simulink model "sampleModel1418"  (R2023a)
settings: Solver=VariableStepAuto  StartTime=0.0  StopTime=10.0  RelTol=1e-3
libraries: hdlsllib x5, simulink x2
settings Model: Creator=user1  LastModifiedBy=user1

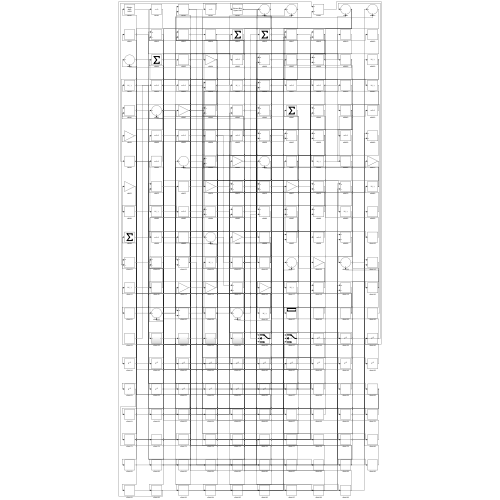
[thumbnail: Simulink's stored preview of the top-level diagram]
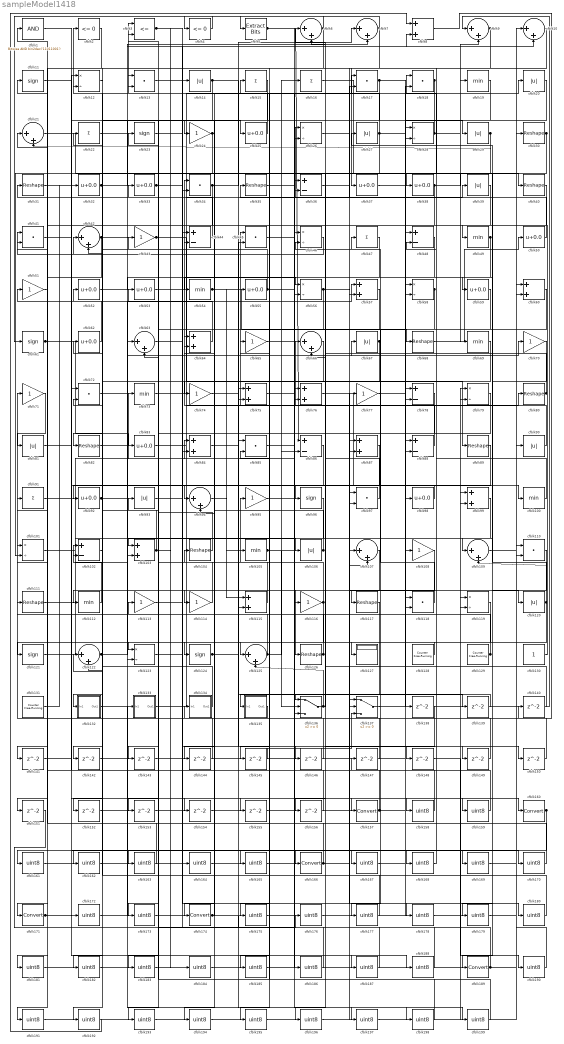
== system sampleModel1418 ==
  cfblk1 : simulink/Logic and Bit Operations/Bitwise Operator  logicop=AND  UseBitMask=on  BitMask=bin2dec('11011001')  BitMaskRealWorld=Stored Integer
      settings: LibrarySourceBlock=|
      | hdlsllib/Logic and Bit
      | Operations/Bitwise
      | Operator
  cfblk{6..7,9..10,21,42,63,66,94,107,109,122,125} (13 alike) : Sum  Inputs=|++
  cfblk{19,49,54,69,73,100,105,112} (8 alike) : MinMax
  cfblk{12,26,28,46,56,58,79,101,119,123} (10 alike) : Product  Inputs=*/  RndMeth=Zero  SaturateOnIntegerOverflow=on
  cfblk{36,44,48,78,86,88,102} (7 alike) : Sum  Inputs=+-
  cfblk{8,57,60,64,75..76,84,87,99,103,115} (11 alike) : Sum
  cfblk{30..31,35,40,68,80,82,89,104,111,117,126} (12 alike) : Reshape
  cfblk{14,20,27,29,39,67,81,90,93,106,120} (11 alike) : Abs  SaturateOnIntegerOverflow=off
  cfblk{24,43,51,65,70..71,74,77,95,108,113..114,116} (13 alike) : Gain
  cfblk{11,23,61,96,121,124} (6 alike) : Signum
  cfblk{13,17..18,34,41,45,72,85,97,110,118} (11 alike) : DotProduct  OutDataTypeStr=Inherit: Inherit via internal rule
  cfblk127 : Display
  cfblk128 : hdlsllib/Sources/Counter Free-Running  NumBits=16  tsamp=-1
  cfblk129 : hdlsllib/Sources/Counter Free-Running  NumBits=16  tsamp=-1
  cfblk130 : Constant  SampleTime=-1
  cfblk131 : hdlsllib/Sources/Counter Free-Running  NumBits=16  tsamp=-1
  cfblk132 : Subsystem
      settings: LibrarySourceBlock=|
      | hdlsllib/Ports &
      | Subsystems/Subsystem
  cfblk133 : Subsystem
      settings: LibrarySourceBlock=|
      | hdlsllib/Ports &
      | Subsystems/Subsystem
  cfblk134 : Subsystem
      settings: LibrarySourceBlock=|
      | hdlsllib/Ports &
      | Subsystems/Subsystem
  cfblk135 : Subsystem
      settings: LibrarySourceBlock=|
      | hdlsllib/Ports &
      | Subsystems/Subsystem
  cfblk136 : Switch  SaturateOnIntegerOverflow=off  InputSameDT=off
  cfblk137 : Switch  SaturateOnIntegerOverflow=off  InputSameDT=off
  cfblk{138..156} (19 alike) : Delay  SampleTime=1
  cfblk{15..16,22,47,91} (5 alike) : Sum  Inputs=+
  cfblk{157,160,166,171,174,189} (6 alike) : DataTypeConversion  SaturateOnIntegerOverflow=off  RndMeth=Floor
  cfblk{158..159,161..165,167..170,172..173,175..188,190..199} (37 alike) : DataTypeConversion  OutDataTypeStr=uint8  SaturateOnIntegerOverflow=off  RndMeth=Floor
  cfblk2 : hdlsllib/Logic and Bit Operations/Compare To Zero  relop=<=  OutDataTypeStr=boolean
  cfblk{25,32..33,37..38,50,52..53,55,59,62,83,92,98} (14 alike) : Bias  Bias=0.0  SaturateOnIntegerOverflow=off
  cfblk3 : RelationalOperator  Operator=<=  OutDataTypeStr=boolean  InputSameDT=off
  cfblk4 : hdlsllib/Logic and Bit Operations/Compare To Zero  relop=<=  OutDataTypeStr=boolean
  cfblk5 : simulink/Logic and Bit Operations/Extract Bits  bitsToExtract=Upper half  numBits=8  bitIdxRange=[0 7]  outScalingMode=Preserve fixed-point scaling
      settings: LibrarySourceBlock=|
      | hdlsllib/Logic and Bit
      | Operations/Extract Bits
  wires:
  cfblk73/1 -> cfblk20/1
  cfblk94/1 -> cfblk115/1
  cfblk68/1 -> cfblk50/1
  cfblk42/1 -> cfblk56/2, cfblk151/1, cfblk170/1
  cfblk130/1 -> cfblk49/1
  cfblk88/1 -> cfblk45/1
  cfblk25/1 -> cfblk2/1
  cfblk106/1 -> cfblk15/1, cfblk13/1
  cfblk54/1 -> cfblk68/1, cfblk105/1
  cfblk83/1 -> cfblk39/1
  cfblk131/1 -> cfblk32/1
  cfblk15/1 -> cfblk82/1
  cfblk121/1 -> cfblk73/1
  cfblk1/1 -> cfblk25/1
  cfblk90/1 -> cfblk34/1
  cfblk93/1 -> cfblk14/1
  cfblk104/1 -> cfblk53/1
  cfblk5/1 -> cfblk86/1, cfblk40/1
  cfblk97/1 -> cfblk6/1
  cfblk135/1(Out1) -> cfblk71/1
  cfblk19/1 -> cfblk74/1
  cfblk101/1 -> cfblk106/1
  cfblk9/1 -> cfblk37/1, cfblk122/2, cfblk57/2
  cfblk18/1 -> cfblk28/2, cfblk103/2
  cfblk12/1 -> cfblk42/2
  cfblk110/1 -> cfblk189/1
  cfblk112/1 -> cfblk102/1
  cfblk80/1 -> cfblk35/1, cfblk47/1
  cfblk28/1 -> cfblk24/1, cfblk9/2
  cfblk117/1 -> cfblk135/1(In1)
  cfblk100/1 -> cfblk18/1
  cfblk61/1 -> cfblk83/1, cfblk187/1
  cfblk34/1 -> cfblk7/1, cfblk123/2
  cfblk57/1 -> cfblk115/2
  cfblk119/1 -> cfblk171/1
  cfblk75/1 -> cfblk160/1
  cfblk7/1 -> cfblk5/1, cfblk152/1
  cfblk108/1 -> cfblk126/1
  cfblk55/1 -> cfblk31/1, cfblk13/2, cfblk159/1
  cfblk70/1 -> cfblk109/1
  cfblk115/1 -> cfblk95/1
  cfblk16/1 -> cfblk98/1
  cfblk133/1(Out1) -> cfblk66/1
  cfblk21/1 -> cfblk69/1
  cfblk96/1 -> cfblk123/1
  cfblk91/1 -> cfblk46/1
  cfblk58/1 -> cfblk124/1, cfblk117/1
  cfblk86/1 -> cfblk125/1
  cfblk52/1 -> cfblk56/1
  cfblk125/1 -> cfblk41/1, cfblk16/1
  cfblk72/1 -> cfblk157/1
  cfblk4/1 -> cfblk61/1
  cfblk48/1 -> cfblk166/1
  cfblk82/1 -> cfblk67/1
  cfblk62/1 -> cfblk11/1
  cfblk56/1 -> cfblk94/1, cfblk150/1
  cfblk124/1 -> cfblk80/1, cfblk194/1
  cfblk118/1 -> cfblk46/2
  cfblk122/1 -> cfblk70/1, cfblk55/1
  cfblk32/1 -> cfblk7/2, cfblk182/1
  cfblk47/1 -> cfblk94/2
  cfblk120/1 -> cfblk27/1, cfblk109/2, cfblk165/1
  cfblk27/1 -> cfblk29/1, cfblk103/1, cfblk3/2, cfblk101/2
  cfblk6/1 -> cfblk4/1, cfblk175/1
  cfblk23/1 -> cfblk34/2
  cfblk71/1 -> cfblk81/1
  cfblk116/1 -> cfblk44/2, cfblk161/1
  cfblk14/1 -> cfblk139/1, cfblk173/1
  cfblk78/1 -> cfblk174/1
  cfblk24/1 -> cfblk132/1(In1), cfblk54/1
  cfblk26/1 -> cfblk120/1
  cfblk50/1 -> cfblk26/1
  cfblk136/1 -> cfblk6/2, cfblk125/2
  cfblk74/1 -> cfblk57/1
  cfblk111/1 -> cfblk63/1
  cfblk33/1 -> cfblk143/1, cfblk167/1
  cfblk2/1 -> cfblk121/1
  cfblk76/1 -> cfblk108/1
  cfblk109/1 -> cfblk30/1
  cfblk92/1 -> cfblk84/1, cfblk112/1
  cfblk98/1 -> cfblk92/1
  cfblk77/1 -> cfblk118/1
  cfblk29/1 -> cfblk116/1, cfblk21/2
  cfblk43/1 -> cfblk89/1, cfblk17/2
  cfblk44/1 -> cfblk12/2
  cfblk103/1 -> cfblk52/1, cfblk184/1
  cfblk123/1 -> cfblk84/2
  cfblk53/1 -> cfblk97/2
  cfblk105/1 -> cfblk26/2, cfblk86/2, cfblk136/2
  cfblk45/1 -> cfblk100/1
  cfblk46/1 -> cfblk41/2
  cfblk126/1 -> cfblk21/1, cfblk101/1
  cfblk67/1 -> cfblk114/1, cfblk145/1
  cfblk22/1 -> cfblk10/2
  cfblk38/1 -> cfblk19/1, cfblk58/2
  cfblk129/1 -> cfblk63/2, cfblk64/1
  cfblk3/1 -> cfblk158/1, cfblk164/1
  cfblk134/1(Out1) -> cfblk102/2
  cfblk49/1 -> cfblk136/1, cfblk185/1
  cfblk10/1 -> cfblk38/1
  cfblk30/1 -> cfblk136/3, cfblk179/1
  cfblk40/1 -> cfblk59/1
  cfblk81/1 -> cfblk96/1
  cfblk114/1 -> cfblk3/1
  cfblk95/1 -> cfblk17/1
  cfblk128/1 -> cfblk127/1
  cfblk64/1 -> cfblk22/1
  cfblk17/1 -> cfblk118/2, cfblk76/2
  cfblk137/1 -> cfblk9/1
  cfblk20/1 -> cfblk88/2
  cfblk13/1 -> cfblk8/2
  cfblk37/1 -> cfblk138/1
  cfblk139/1 -> cfblk137/2
  cfblk8/1 -> cfblk140/1
  cfblk140/1 -> cfblk66/2
  cfblk51/1 -> cfblk141/1
  cfblk102/1 -> cfblk142/1
  cfblk142/1 -> cfblk28/1
  cfblk143/1 -> cfblk45/2
  cfblk69/1 -> cfblk144/1
  cfblk144/1 -> cfblk12/1
  cfblk145/1 -> cfblk137/3
  cfblk63/1 -> cfblk146/1
  cfblk146/1 -> cfblk76/1
  cfblk147/1 -> cfblk1/1
  cfblk35/1 -> cfblk148/1
  cfblk84/1 -> cfblk149/1
  cfblk149/1 -> cfblk42/1
  cfblk150/1 -> cfblk122/1
  cfblk152/1 -> cfblk88/1
  cfblk59/1 -> cfblk153/1
  cfblk11/1 -> cfblk154/1
  cfblk154/1 -> cfblk97/1
  cfblk31/1 -> cfblk155/1
  cfblk155/1 -> cfblk18/2
  cfblk89/1 -> cfblk156/1
  cfblk156/1 -> cfblk43/1
  cfblk157/1 -> cfblk147/1, cfblk111/1
  cfblk158/1 -> cfblk72/1
  cfblk159/1 -> cfblk72/2
  cfblk160/1 -> cfblk191/1, cfblk193/1
  cfblk161/1 -> cfblk75/1
  cfblk66/1 -> cfblk162/1
  cfblk162/1 -> cfblk75/2
  cfblk87/1 -> cfblk163/1
  cfblk163/1 -> cfblk91/1
  cfblk164/1 -> cfblk87/1
  cfblk165/1 -> cfblk87/2
  cfblk166/1 -> cfblk134/1(In1), cfblk51/1
  cfblk167/1 -> cfblk48/1
  cfblk41/1 -> cfblk168/1
  cfblk168/1 -> cfblk48/2
  cfblk113/1 -> cfblk169/1
  cfblk169/1 -> cfblk10/1
  cfblk170/1 -> cfblk113/1
  cfblk171/1 -> cfblk58/1, cfblk133/1(In1), cfblk188/1
  cfblk141/1 -> cfblk172/1
  cfblk172/1 -> cfblk119/1
  cfblk173/1 -> cfblk119/2
  cfblk174/1 -> cfblk64/2, cfblk77/1, cfblk199/1
  cfblk175/1 -> cfblk78/1
  cfblk151/1 -> cfblk176/1
  cfblk176/1 -> cfblk78/2
  cfblk60/1 -> cfblk177/1
  cfblk177/1 -> cfblk104/1
  cfblk153/1 -> cfblk178/1
  cfblk178/1 -> cfblk60/1
  cfblk179/1 -> cfblk60/2
  cfblk36/1 -> cfblk180/1
  cfblk180/1 -> cfblk62/1
  cfblk39/1 -> cfblk181/1
  cfblk181/1 -> cfblk36/1
  cfblk182/1 -> cfblk36/2
  cfblk79/1 -> cfblk183/1
  cfblk183/1 -> cfblk90/1
  cfblk184/1 -> cfblk79/1
  cfblk185/1 -> cfblk79/2
  cfblk85/1 -> cfblk186/1
  cfblk186/1 -> cfblk23/1
  cfblk187/1 -> cfblk85/1
  cfblk188/1 -> cfblk85/2
  cfblk189/1 -> cfblk44/1, cfblk33/1
  cfblk148/1 -> cfblk190/1
  cfblk190/1 -> cfblk110/1
  cfblk191/1 -> cfblk110/2
  cfblk107/1 -> cfblk192/1
  cfblk192/1 -> cfblk8/1
  cfblk193/1 -> cfblk107/1
  cfblk194/1 -> cfblk107/2
  cfblk99/1 -> cfblk195/1
  cfblk195/1 -> cfblk137/1
  cfblk138/1 -> cfblk196/1
  cfblk196/1 -> cfblk99/1
  cfblk132/1(Out1) -> cfblk197/1
  cfblk197/1 -> cfblk99/2
  cfblk65/1 -> cfblk198/1
  cfblk198/1 -> cfblk93/1
  cfblk199/1 -> cfblk65/1

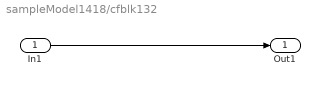
== system sampleModel1418/cfblk132 ==
  In1 : Inport
  Out1 : Outport
  wires:
  In1/1 -> Out1/1

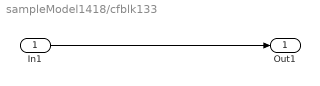
== system sampleModel1418/cfblk133 ==
  In1 : Inport
  Out1 : Outport
  wires:
  In1/1 -> Out1/1

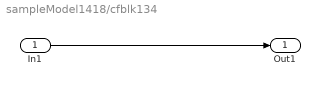
== system sampleModel1418/cfblk134 ==
  In1 : Inport
  Out1 : Outport
  wires:
  In1/1 -> Out1/1

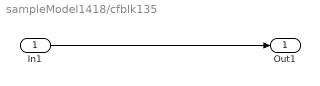
== system sampleModel1418/cfblk135 ==
  In1 : Inport
  Out1 : Outport
  wires:
  In1/1 -> Out1/1
